simulink model "ship"  (R2016a)
settings: Solver=ode8  StartTime=0.0  StopTime=1200  FixedStep=0.005  RelTol=1e-3
settings Model: Creator=bernd  LastModifiedBy=bernd

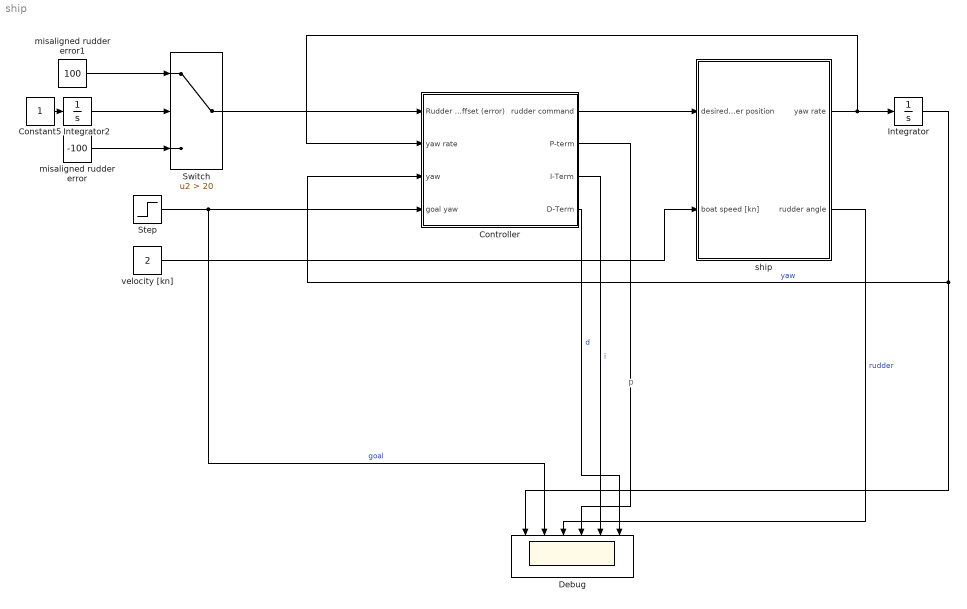
== system ship ==
  note: p
  Constant5 : Constant
  Controller : Subsystem
  Debug : Scope  NumInputPorts=6
  Integrator : Integrator
  Integrator2 : Integrator
  Step : Step  Time=20  After=50  SampleTime=0
  Switch : Switch  Criteria=u2 > Threshold  Threshold=20
  misaligned rudder error : Constant  Value=-100
  misaligned rudder error1 : Constant  Value=100
  ship : Subsystem
  velocity [kn] : Constant  Value=2
  wires:
  Step/1 -> Debug/2, Controller/4(goal yaw)  "goal"
  Integrator/1 -> Controller/3(yaw), Debug/1  "yaw"
  velocity [kn]/1 -> ship/2("boat speed [kn] ")
  ship/2("rudder angle ") -> Debug/3  "rudder"
  ship/1(yaw rate) -> Controller/2(yaw rate), Integrator/1
  Controller/1(rudder command) -> ship/1(desired rudder position)
  Controller/2(P-term) -> Debug/4
  Controller/3(I-Term) -> Debug/5  "i"
  Controller/4(D-Term) -> Debug/6  "d"
  Switch/1 -> Controller/1("Rudder offset (error) ")
  misaligned rudder error/1 -> Switch/3
  Integrator2/1 -> Switch/2
  misaligned rudder error1/1 -> Switch/1
  Constant5/1 -> Integrator2/1

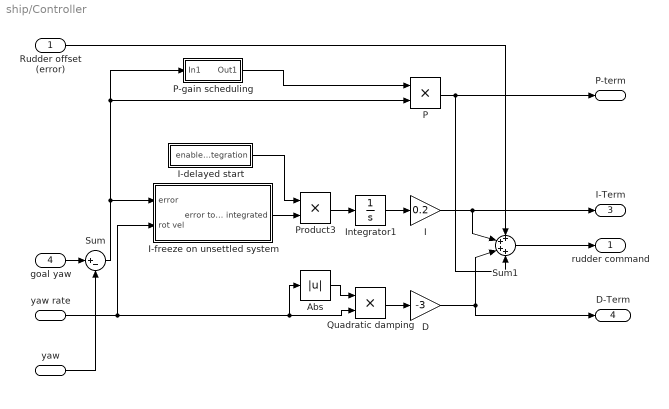
== system ship/Controller ==
  "Rudder offset (error) " : Inport
  yaw rate : Inport  Port=2
  yaw : Inport  Port=3
  goal yaw : Inport  Port=4
  Abs : Abs
  D : Gain  Gain=-3
  I : Gain  Gain=0.2
  I-delayed start : Subsystem
  I-freeze on unsettled system : Subsystem
  Integrator1 : Integrator
  P : Product
  P-gain scheduling : Subsystem
  Product3 : Product
  Quadratic damping : Product
  Sum : Sum  Inputs=|+-
  Sum1 : Sum  Inputs=++++
  rudder command : Outport
  P-term : Outport  Port=2
  I-Term : Outport  Port=3
  D-Term : Outport  Port=4
  wires:
  goal yaw/1 -> Sum/1
  Quadratic damping/1 -> D/1
  P-gain scheduling/1(Out1) -> P/1
  I-freeze on unsettled system/1(error to be integrated) -> Product3/2
  D/1 -> Sum1/3, D-Term/1
  I-delayed start/1(enable integration) -> Product3/1
  Sum1/1 -> rudder command/1
  yaw/1 -> Sum/2
  "Rudder offset (error) "/1 -> Sum1/1
  I/1 -> Sum1/2, I-Term/1
  yaw rate/1 -> I-freeze on unsettled system/2(rot vel), Abs/1, Quadratic damping/2
  Integrator1/1 -> I/1
  P/1 -> P-term/1, Sum1/4
  Abs/1 -> Quadratic damping/1
  Product3/1 -> Integrator1/1
  Sum/1 -> P-gain scheduling/1(In1), P/2, I-freeze on unsettled system/1(error)

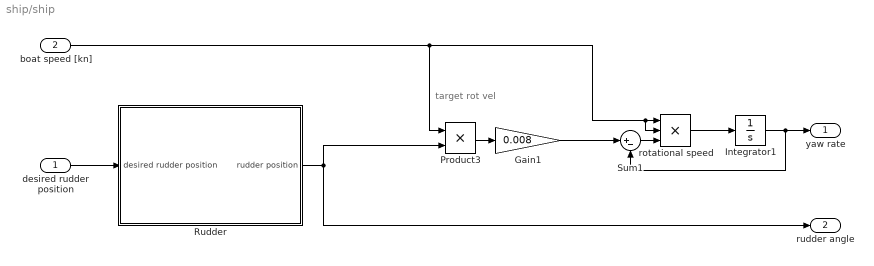
== system ship/ship ==
  note: target rot vel
  desired rudder position : Inport
  "boat speed [kn] " : Inport  Port=2
  Gain1 : Gain  Gain=0.008
  Integrator1 : Integrator
  Product3 : Product
  "Rudder " : Subsystem
  Sum1 : Sum  Inputs=|+-
  rotational speed : Product  Inputs=3
  yaw rate : Outport
  "rudder angle " : Outport  Port=2
  wires:
  Sum1/1 -> rotational speed/3
  rotational speed/1 -> Integrator1/1
  Integrator1/1 -> yaw rate/1, Sum1/2
  "boat speed [kn] "/1 -> Product3/1, rotational speed/2, rotational speed/1
  desired rudder position/1 -> "Rudder "/1("desired rudder position ")
  Gain1/1 -> Sum1/1
  Product3/1 -> Gain1/1
  "Rudder "/1(rudder position) -> Product3/2, "rudder angle "/1

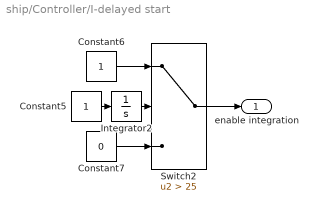
== system ship/Controller/I-delayed start ==
  Constant5 : Constant
  Constant6 : Constant
  Constant7 : Constant  Value=0
  Integrator2 : Integrator
  Switch2 : Switch  Criteria=u2 > Threshold  Threshold=25
  enable integration : Outport
  wires:
  Constant5/1 -> Integrator2/1
  Integrator2/1 -> Switch2/2
  Constant6/1 -> Switch2/1
  Constant7/1 -> Switch2/3
  Switch2/1 -> enable integration/1

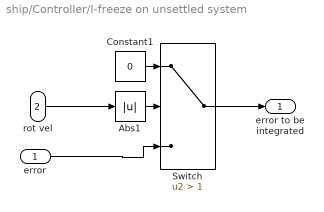
== system ship/Controller/I-freeze on unsettled system ==
  error : Inport
  rot vel : Inport  Port=2
  Abs1 : Abs
  Constant1 : Constant  Value=0
  Switch : Switch  Criteria=u2 > Threshold  Threshold=1
  error to be integrated : Outport
  wires:
  Abs1/1 -> Switch/2
  Constant1/1 -> Switch/1
  Switch/1 -> error to be integrated/1
  rot vel/1 -> Abs1/1
  error/1 -> Switch/3

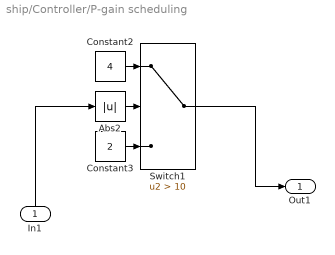
== system ship/Controller/P-gain scheduling ==
  In1 : Inport
  Abs2 : Abs
  Constant2 : Constant  Value=4
  Constant3 : Constant  Value=2
  Switch1 : Switch  Criteria=u2 > Threshold  Threshold=10
  Out1 : Outport
  wires:
  In1/1 -> Abs2/1
  Constant3/1 -> Switch1/3
  Abs2/1 -> Switch1/2
  Switch1/1 -> Out1/1
  Constant2/1 -> Switch1/1

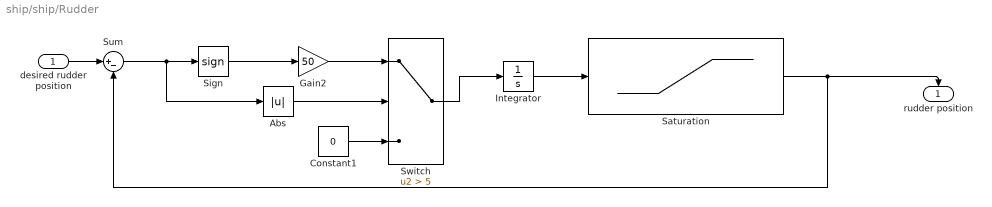
== system ship/ship/Rudder  ==
  "desired rudder position " : Inport
  Abs : Abs
  Constant1 : Constant  Value=0
  Gain2 : Gain  Gain=50
  Integrator : Integrator
  Saturation : Saturate  UpperLimit=250  LowerLimit=-250
  Sign : Signum
  Sum : Sum  Inputs=|+-
  Switch : Switch  Criteria=u2 > Threshold  Threshold=5
  rudder position : Outport
  wires:
  Saturation/1 -> Sum/2, rudder position/1
  Abs/1 -> Switch/2
  Sum/1 -> Abs/1, Sign/1
  "desired rudder position "/1 -> Sum/1
  Constant1/1 -> Switch/3
  Gain2/1 -> Switch/1
  Sign/1 -> Gain2/1
  Integrator/1 -> Saturation/1
  Switch/1 -> Integrator/1
